simulink model "ex77"  (R2023b)
settings: Solver=VariableStepAuto  StartTime=0.0  StopTime=10.0  RelTol=1e-3
settings Model: Creator=sorin  LastModifiedBy=sorin

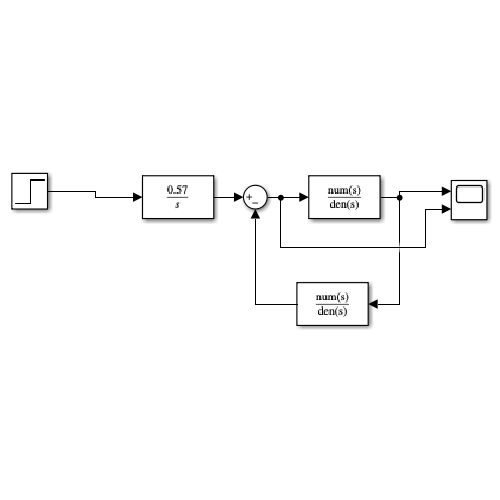
[thumbnail: Simulink's stored preview of the top-level diagram]
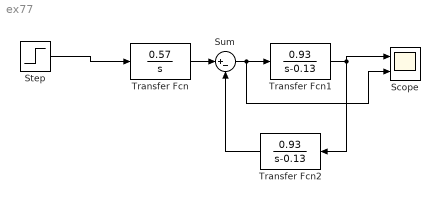
== system ex77 ==
  Scope : Scope  NumInputPorts=2
  Step : Step  After=20  SampleTime=0
  Sum : Sum  Inputs=|+-
  Transfer Fcn : TransferFcn  Numerator=[0.57]  Denominator=[1 0]
  Transfer Fcn1 : TransferFcn  Numerator=[0.93]  Denominator=[1 -0.13]
  Transfer Fcn2 : TransferFcn  Numerator=[0.93]  Denominator=[1 -0.13]
  wires:
  Transfer Fcn1/1 -> Transfer Fcn2/1, Scope/1
  Step/1 -> Transfer Fcn/1
  Transfer Fcn/1 -> Sum/1
  Sum/1 -> Scope/2, Transfer Fcn1/1
  Transfer Fcn2/1 -> Sum/2
